simulink model "dynamic_friction_2015"  (R2015a)
settings: Solver=ode4  StartTime=0.0  StopTime=inf  FixedStep=0.001  RelTol=1e-3
libraries: PoliArd x6
settings Model: CovHtmlReporting=off  ExtModeTrigDuration=2  Creator=User  LastModifiedBy=User
settings OptimizationCC: OptimizeModelRefInitCode=on  LifeSpan=1
settings DebuggingCC: UnderspecifiedInitializationDetection=Classic  MergeDetectMultiDrivingBlocksExec=none
settings HardwareCC: ProdLargestAtomicInteger=Long  ProdLargestAtomicFloat=Double  ProdEndianess=LittleEndian  ProdHWDeviceType=ARM Compatible->ARM Cortex
settings RTWCC: SystemTargetFile=realtime.tlc  GenerateMakefile=off  TemplateMakefile=realtime.tmf  Description=Run on Target Hardware  RTWVerbose=off
settings ERTTargetCC: CombineOutputUpdateFcns=off  ExtModeTransport=3  ExtModeMexFile=ext_serial_win32_comm_rtt  ExtModeMexArgs=0 1 9600  InlinedParameterPlacement=Hierarchical  ERTSrcFileBannerTemplate=realtime_code_template.cgt  ERTHdrFileBannerTemplate=realtime_code_template.cgt  ERTDataSrcFileTemplate=realtime_code_template.cgt  ERTDataHdrFileTemplate=realtime_code_template.cgt  ERTCustomFileTemplate=realtime_file_process.tlc

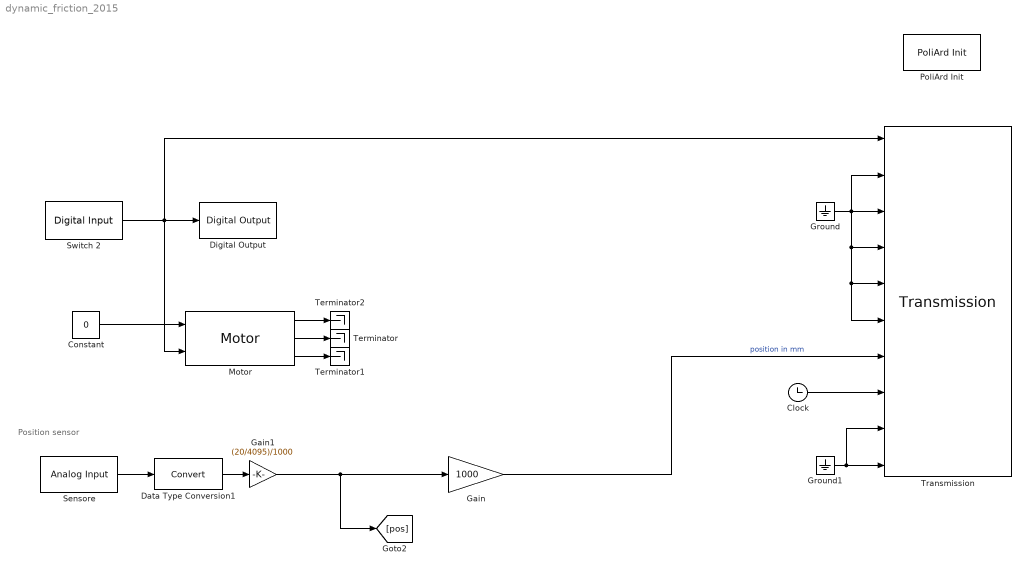
== system dynamic_friction_2015 ==
  note: Position sensor
  Clock : Clock
  Constant : Constant  Value=0
  Data Type Conversion1 : DataTypeConversion
  Digital Output : PoliArd/Digital Output  DO_pin=1
  Gain : Gain  Gain=1000
  Gain1 : Gain  Gain=(20/4095)/1000
  Ground : Ground
  Ground1 : Ground
  Motor : PoliArd/Motor  MotorID=2  DC_bus_mask=24  dt_mot=-1
  PoliArd Init : PoliArd/PoliArd Init
  Sensore : PoliArd/Analog Input  AIpin_mask=2  AIsample=-1
  Switch 2 : PoliArd/Digital Input  DI_pin=2  DIsample=-1
  Terminator : Terminator
  Terminator1 : Terminator
  Terminator2 : Terminator
  Transmission : PoliArd/Transmission  sample_freq=1000  sig_to_send=6
  wires:
  Gain1/1 -> [pos], Gain/1
  Data Type Conversion1/1 -> Gain1/1
  Switch 2/1 -> Transmission/1, Digital Output/1, Motor/2
  Ground/1 -> Transmission/2, Transmission/6, Transmission/5, Transmission/4, Transmission/3
  Sensore/1 -> Data Type Conversion1/1
  Clock/1 -> Transmission/8
  Gain/1 -> Transmission/7  "position in mm"
  Motor/2 -> Terminator/1
  Motor/3 -> Terminator1/1
  Ground1/1 -> Transmission/9, Transmission/10
  Constant/1 -> Motor/1
  Motor/1 -> Terminator2/1
